simulink model "RAPID_0_ADCS_Model_practice"  (R2024b)
settings: Solver=VariableStepAuto  StartTime=0.0  StopTime=10.0  RelTol=1e-3
undefined symbols (not defined in the file): I
settings Model: Creator=aditi  LastModifiedBy=aditi

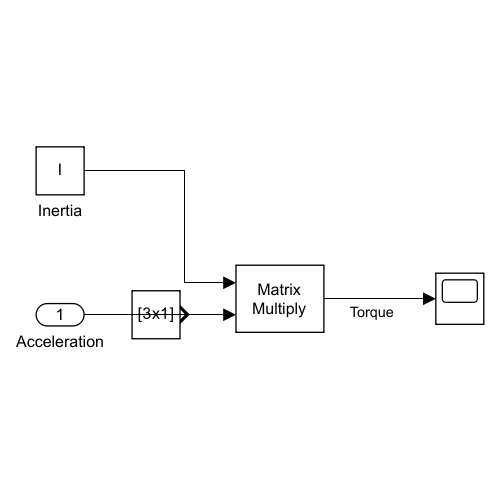
[thumbnail: Simulink's stored preview of the top-level diagram]
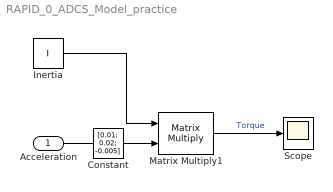
== system RAPID_0_ADCS_Model_practice ==
  Acceleration : Inport  PortDimensions=[3 1]
  Constant : Constant  Value=[0.01; 0.02; -0.005]
  Inertia : Constant  Value=I  VectorParams1D=off
  Matrix Multiply1 : Product  Multiplication=Matrix(*)
  Scope : Scope
  wires:
  Inertia/1 -> Matrix Multiply1/1
  Acceleration/1 -> Matrix Multiply1/2
  Matrix Multiply1/1 -> Scope/1  "Torque"
